simulink model "psm_svpwm_nonlinear_ctrl"  (R2026a)
settings: Solver=ode23tb  StopTime=simlength  FixedStep=tc  MaxStep=tc
values from neighbouring files (symbols this model uses):
  CTRPIFF_CLIP_RELEASE = 0.001    [init_model.m]
  dead_time_INV = 3e-6    (= 3e-06)    [init_model.m]
  emf_fb_p = 0.2    [init_model.m]
  emf_fb_p_ccaller_1 = emf_fb_p    (= 0.2)    [init_model.m]
  emf_fb_p_ccaller_2 = emf_fb_p    (= 0.2)    [init_model.m]
  emf_p = emf_fb_p*4/10    (= 0.08)    [init_model.m]
  emf_p_ccaller_1 = emf_fb_p_ccaller_1*4/10    (= 0.08)    [init_model.m]
  emf_p_ccaller_2 = emf_fb_p_ccaller_2*4/10    (= 0.08)    [init_model.m]
  fPWM_INV = fPWM_AFE    (= 5000)    [init_model.m]
  g0_10Hz = fcut_10Hz_flt * ts_afe * 2*pi    (= 0.0125663706144)    [init_model.m]
  g0_1Hz = fcut_1Hz_flt * ts_afe * 2*pi    (= 0.00125663706144)    [init_model.m]
  g1_10Hz = 1 - g0_10Hz    (= 0.987433629386)    [init_model.m]
  g1_1Hz = 1 - g0_1Hz    (= 0.998743362939)    [init_model.m]
  id_lim = 0.35    [init_model.m]
  inv_m_scale = motorc_m_scale    [init_model.m]
  iq_lim = 1.4    [init_model.m]
  kg = Kobs(1)    [init_model.m]
  ki_align = 0.1    [init_model.m]
  ki_i = 18    [init_model.m]
  ki_w = 32    [init_model.m]
  kp_align = 0.6    [init_model.m]
  kp_i = 0.25    [init_model.m]
  kp_w = 2    [init_model.m]
  kw = Kobs(2)    [init_model.m]
  lim_down_align = -0.2    [init_model.m]
  lim_up_align = 0.2    [init_model.m]
  number_of_modules = 1    [init_model.m]
  omega_m_sim = omega_m_bez    [init_model.m]
  simlength = 2    [init_model.m]
  tc = ts_afe/100    (= 2e-06)    [init_model.m]
  time_gain_afe_module_1 = 1.0    (= 1)    [init_model.m]
  time_gain_inv_module_2 = 1.0    (= 1)    [init_model.m]
  time_start_motor_control = 0.025    [init_model.m]
  ts_inv = 1/fPWM_INV    (= 0.0002)    [init_model.m]
undefined symbols (not defined in the file or in its folder): ibez, La, Lb, Ld_norm, Lq_norm, Ls_norm, magnitude, omega_bez, omega_m_bez, psi_bez, psi_m, psi_m_norm, rpm_base, rpm_bez, Rs, Rs_norm, tau_bez, torque_base, ubez
libraries: fl_lib x24, nesl_utility x11, cstblocks_lti x2, single_phase_pwm_modulator x1, pi_ctrl x1, threephase_inductor_lib x1, simple_flexible_shaft x1, permanent_magnet_synchronous_machine x1
(part 2 of 3)

== system psm_svpwm_nonlinear_ctrl/inv_psm_mod1/inverter_ctrl/inverter_control/current_ctrl/bemf_observer ==
  ialpha_pu : Inport
  ibeta_pu : Inport  Port=2
  ualpha_pu : Inport  Port=3
  ubeta_pu : Inport  Port=4
  udc_pu : Inport  Port=5
  BEMF Observer simulink/Ccaller mod1 : Scope  NumInputPorts=2
      settings: ActiveDisplayYMinimum=-0.23480320261212159  ActiveDisplayYMaximum=2.113226231053849
  Mux : Mux  Inputs=3
  Mux1 : Mux  Inputs=3
  Variant Source : VariantSource  VariantControls={use_observer_from_simulink_module_1 == 1, use_observer_from_ccaller_module_1 == 1}
  Variant Source1 : VariantSource  VariantControls={use_observer_from_simulink_module_1 == 1, use_observer_from_ccaller_module_1 == 1}
  bemf_observer : Subsystem  Commented=on
  bemf_observer_ccaller : Subsystem
  nonlinear_observer : Subsystem
  tag scope: omega_hat_pu_mod1=scoped, phase_hat_mod1=scoped
  wires:
  ialpha_pu/1 -> bemf_observer_ccaller/1(ialpha_pu), nonlinear_observer/1(ialpha_pu)
  ibeta_pu/1 -> bemf_observer_ccaller/2(ibeta_pu), nonlinear_observer/2(ibeta_pu)
  Mux/1 -> BEMF Observer simulink/Ccaller mod1/1
  Mux1/1 -> BEMF Observer simulink/Ccaller mod1/2
  ualpha_pu/1 -> bemf_observer_ccaller/3(ualpha_pu), nonlinear_observer/3(ualpha_pu)
  ubeta_pu/1 -> bemf_observer_ccaller/4(ubeta_pu), nonlinear_observer/4(ubeta_pu)
  bemf_observer_ccaller/2(theta_hat) -> Mux1/2, Variant Source1/2  "theta_hat_code"
  bemf_observer_ccaller/1(omega_pu) -> Mux/2, Variant Source/2  "omega_pu_code"
  Variant Source1/1 -> [phase_hat_mod1]
  Variant Source/1 -> [omega_hat_pu_mod1]
  udc_pu/1 -> bemf_observer_ccaller/5(udc_pu), nonlinear_observer/5(udc_pu)
  [omega_pu_psm] -> Mux/3  "omega_pu_psm_encoder"
  [phased_psm] -> Mux1/3  "phase_psm_encoder"
  [theta_z_hat] -> Variant Source1/1
  [omega_z_pu_hat] -> Variant Source/1
  [omega_z_pu_hat] -> Mux/1
  [theta_z_hat] -> Mux1/1

== system psm_svpwm_nonlinear_ctrl/inv_psm_mod1/inverter_ctrl/inverter_control/current_ctrl/current_ctrl ==
  iq_ref : Inport
  udc_pu : Inport  Port=2
  MTPA _mod1 : Subsystem
  Sqrt : Sqrt
  Square : Math  Operator=square
  Square1 : Math  Operator=square
  Sum : Sum  Inputs=|++
  dq_pi_with_vector_antiwindup mod1 : Subsystem
  id_ref _mod1 : Subsystem
      settings: PortSchema="{\"entries\":[{\"content\":{\"sides\":[{\"content\":{},\"type\":\"ConnectorPlacement.EquallySpacedRectSide\",\"uuid\":\"42af5d69-f0eb-42c6-9e03-28c1d0757323\"},{\"content\":{\"connectorIds\":[\"Out1\"],\"side\":\"RIGHT\"},\"type\":\"ConnectorPlacement.EquallySpacedRectSide\",\"uuid\":\"dd68a9f9-d15f-4e57-9d9e-130889a7b90c\"},{\"content\":{\"connectorIds\":[\"In1\"],\"side\":\"TOP\"},\"type\":\"ConnectorPlacement.EquallySpacedRectSide\",\"uuid\":\"68c797a2-8439-4b8d-8368-b7485adf0676\"}]},\"type\":\"ConnectorPlacement.EquallySpacedConnector\",\"uuid\":\"693c5f1c-0580-4626-8f13-b27865dfb3ac\"}],\"packageUris\":[\"http://schema.mathworks.com/mf0/Connector/R2020b\"],\"version\":\"1.0\"}"
  idref/id mod1 : Scope  NumInputPorts=2
      settings: ActiveDisplayYMinimum=-1.4397848868479775  ActiveDisplayYMaximum=0.32158973081029762
  iqref/iq mod1 : Scope  NumInputPorts=2
      settings: ActiveDisplayYMinimum=-1.2112726866098484  ActiveDisplayYMaximum=0.690933447736122  DataLoggingVariableName=ScopeData2
  output voltage transformation : Subsystem
  tag scope: id_pu_ref_mod1=scoped, iq_pu_ref_mod1=scoped, u_mot_pu_mod1=scoped, ud_pu_mod1=scoped, uq_pu_mod1=scoped
  wires:
  [iq_pu_mod1] -> iqref/iq mod1/2, dq_pi_with_vector_antiwindup mod1/4(iq)  "iq"
  [id_pu_mod1] -> idref/id mod1/2, dq_pi_with_vector_antiwindup mod1/2(id)  "id"
  MTPA _mod1/1(Id_ref_mtpa) -> id_ref _mod1/1(id_mtpa), [id_pu_ref_mod1]  "id_ref"
  iq_ref/1 -> MTPA _mod1/1(iq_ref), iqref/iq mod1/1, dq_pi_with_vector_antiwindup mod1/3(iq_ref), [iq_pu_ref_mod1]  "iq_ref"
  dq_pi_with_vector_antiwindup mod1/1(ctrl_d_u) -> [ud_pu_mod1], Square1/1
  dq_pi_with_vector_antiwindup mod1/2(ctrl_q_u) -> [uq_pu_mod1], Square/1
  Square/1 -> Sum/1
  Sum/1 -> Sqrt/1
  Square1/1 -> Sum/2
  Sqrt/1 -> [u_mot_pu_mod1]
  id_ref _mod1/1(id_ref) -> idref/id mod1/1, dq_pi_with_vector_antiwindup mod1/1(id_ref)
  udc_pu/1 -> dq_pi_with_vector_antiwindup mod1/5(udc_pu)

== system psm_svpwm_nonlinear_ctrl/inv_psm_mod1/inverter_ctrl/inverter_control/current_ctrl/current_transformation ==
  Demux : Demux  Outputs=3
  alphabeta2dq : MATLAB Function  TreatAsAtomicUnit=on
  uvw2alphabeta : MATLAB Function  TreatAsAtomicUnit=on
  tag scope: ialpha_pu_mod1=scoped, ibeta_pu_mod1=scoped, id_pu_mod1=scoped, iq_pu_mod1=scoped
  wires:
  alphabeta2dq/2(q) -> [iq_pu_mod1]  "iq_pu"
  alphabeta2dq/1(d) -> [id_pu_mod1]  "id_pu"
  uvw2alphabeta/2(beta) -> alphabeta2dq/2(beta), [ibeta_pu_mod1]  "ibeta_pu"
  uvw2alphabeta/1(alpha) -> [ialpha_pu_mod1], alphabeta2dq/1(alpha)  "ialpha_pu"
  [motor_phase_ctrl_mod1] -> alphabeta2dq/3(gamma)
  Demux/3 -> uvw2alphabeta/3(w)  "iw"
  Demux/2 -> uvw2alphabeta/2(v)  "iv"
  Demux/1 -> uvw2alphabeta/1(u)  "iu"
  [isd_uvw_inv_mod1] -> Demux/1

== system psm_svpwm_nonlinear_ctrl/inv_psm_mod1/inverter_ctrl/inverter_control/encoder-sensorless-switch/double_integrator_observer ==
  theta_psm : Inport
  Dead Zone : DeadZone  LowerValue=-0.01  UpperValue=0.01
  Gain : Gain  Gain=kw
  Gain1 : Gain  Gain=kg
  Gain2 : Gain  Gain=omega_bez
  Gain3 : Gain  Gain=1/omega_bez
  Gain5 : Gain  Gain=ts_inv
  Sum : Sum  Inputs=-+|
  Sum1 : Sum  Inputs=|++
  Sum2 : Sum  Inputs=|++
  Sum8 : Sum  Inputs=++|
  Unit Delay1 : UnitDelay  InitialCondition=pi  SampleTime=-1
  Unit Delay2 : UnitDelay  SampleTime=-1
  bounder1 : MATLAB Function  TreatAsAtomicUnit=on
  bounder2 : MATLAB Function  TreatAsAtomicUnit=on
  phase_psm_hat : Outport  VectorParamsAs1DForOutWhenUnconnected=off
  omega_pu_psm_hat : Outport  Port=2  VectorParamsAs1DForOutWhenUnconnected=off
  wires:
  Gain1/1 -> Sum2/1
  theta_psm/1 -> Sum/2
  Sum8/1 -> Unit Delay1/1
  Unit Delay1/1 -> bounder2/1(u)
  Sum1/1 -> Unit Delay2/1
  Gain/1 -> Gain3/1
  Unit Delay2/1 -> omega_pu_psm_hat/1, Sum1/2, Gain5/1
  Sum2/1 -> Sum8/2
  bounder2/1(y) -> Sum2/2, phase_psm_hat/1, Sum/1  "phase_hat"
  bounder1/1(y) -> Gain1/1, Gain/1
  Gain2/1 -> Sum8/1
  Gain3/1 -> Sum1/1
  Gain5/1 -> Gain2/1
  Sum/1 -> bounder1/1(u)

== system psm_svpwm_nonlinear_ctrl/inv_psm_mod1/inverter_ctrl/inverter_control/is inv quantizzation and one step delay/is inv quantizzation and one step delay ==
  is_u_pu : Inport
  is_v_pu : Inport  Port=2
  is_w_pu : Inport  Port=3
  Gain3 : Gain  Gain=-1
  Gain4 : Gain  Gain=-1
  Gain5 : Gain  Gain=-1
  Quantizer : Quantizer  QuantizationInterval=adc_quantization
  Quantizer1 : Quantizer  QuantizationInterval=adc_quantization
  Quantizer2 : Quantizer  QuantizationInterval=adc_quantization
  Unit Delay : UnitDelay  SampleTime=-1
  Unit Delay1 : UnitDelay  SampleTime=-1
  Unit Delay2 : UnitDelay  SampleTime=-1
  Zero-Order Hold : ZeroOrderHold  SampleTime=-1
  Zero-Order Hold1 : ZeroOrderHold  SampleTime=-1
  Zero-Order Hold2 : ZeroOrderHold  SampleTime=-1
  isd_u_pu : Outport
  isd_v_pu : Outport  Port=2
  isd_w_pu : Outport  Port=3
  wires:
  Unit Delay/1 -> Gain3/1
  Unit Delay1/1 -> Gain4/1
  Unit Delay2/1 -> Gain5/1
  Quantizer/1 -> Unit Delay/1
  Quantizer1/1 -> Unit Delay1/1
  Quantizer2/1 -> Unit Delay2/1
  is_u_pu/1 -> Zero-Order Hold/1
  is_v_pu/1 -> Zero-Order Hold1/1
  is_w_pu/1 -> Zero-Order Hold2/1
  Gain3/1 -> isd_u_pu/1
  Gain4/1 -> isd_v_pu/1
  Gain5/1 -> isd_w_pu/1
  Zero-Order Hold/1 -> Quantizer/1
  Zero-Order Hold1/1 -> Quantizer1/1
  Zero-Order Hold2/1 -> Quantizer2/1

== system psm_svpwm_nonlinear_ctrl/inv_psm_mod1/inverter_ctrl/inverter_control/omega_pu/flt ==
  input : Inport
  Gain3 : Gain  Gain=g1_10Hz
  Gain6 : Gain  Gain=g0_10Hz
  Sum : Sum  Inputs=|++
  Unit Delay1 : UnitDelay  SampleTime=-1
  output : Outport  VectorParamsAs1DForOutWhenUnconnected=off
  wires:
  Gain6/1 -> Sum/1
  input/1 -> Gain6/1
  Unit Delay1/1 -> Gain3/1
  Gain3/1 -> Sum/2
  Sum/1 -> Unit Delay1/1, output/1

== system psm_svpwm_nonlinear_ctrl/inv_psm_mod1/inverter_ctrl/inverter_control/phase_compensation_1/alignment_ctrl ==
  local_time : Inport
  master_time : Inport  Port=2
  Constant : Constant  Value=0
  Gain : Gain  Gain=-1
  Sum : Sum  Inputs=|+-
  pi : Subsystem  mask{kp=kp_align, ki=ki_align, lim_up=lim_up_align, lim_down=lim_down_align}
      mask prompts: ki "ki*ts"
      mask Display:
      | disp('pi()');
      | port_label('input', 1, 'u_ref');
      | port_label('input', 2, 'u');
      | port_label('output', 1, 'y');
  dp : Outport
  wires:
  master_time/1 -> Sum/1
  Sum/1 -> Gain/1
  Constant/1 -> pi/1(u_ref)
  local_time/1 -> Sum/2
  Gain/1 -> pi/2(u)
  pi/1(y) -> dp/1

== system psm_svpwm_nonlinear_ctrl/inv_psm_mod1/inverter_ctrl/inverter_control/speed_reference_generator/flt ==
  input : Inport
  Gain3 : Gain  Gain=g1_1Hz
  Gain6 : Gain  Gain=g0_1Hz
  Sum : Sum  Inputs=|++
  Unit Delay1 : UnitDelay  SampleTime=-1
  output : Outport  VectorParamsAs1DForOutWhenUnconnected=off
  wires:
  Gain6/1 -> Sum/1
  input/1 -> Gain6/1
  Unit Delay1/1 -> Gain3/1
  Gain3/1 -> Sum/2
  Sum/1 -> Unit Delay1/1, output/1

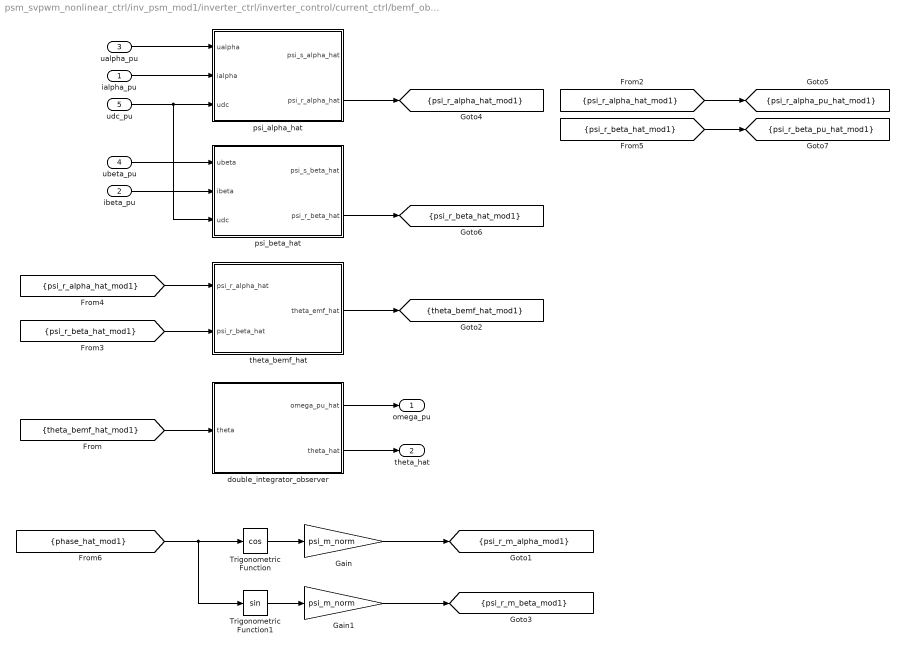
== system psm_svpwm_nonlinear_ctrl/inv_psm_mod1/inverter_ctrl/inverter_control/current_ctrl/bemf_observer/bemf_observer ==
  ialpha_pu : Inport
  ibeta_pu : Inport  Port=2
  ualpha_pu : Inport  Port=3
  ubeta_pu : Inport  Port=4
  udc_pu : Inport  Port=5
  Gain : Gain  Gain=psi_m_norm
  Gain1 : Gain  Gain=psi_m_norm
  Trigonometric Function : Trigonometry  Operator=cos
  Trigonometric Function1 : Trigonometry
  double_integrator_observer : Subsystem
  psi_alpha_hat : Subsystem
  psi_beta_hat : Subsystem
  theta_bemf_hat : Subsystem
  omega_pu : Outport
  theta_hat : Outport  Port=2
  tag scope: psi_r_alpha_hat_mod1=scoped, psi_r_alpha_pu_hat_mod1=scoped, psi_r_beta_hat_mod1=scoped, psi_r_beta_pu_hat_mod1=scoped, psi_r_m_alpha_mod1=scoped, psi_r_m_beta_mod1=scoped, theta_bemf_hat_mod1=scoped
  wires:
  Trigonometric Function/1 -> Gain/1
  Trigonometric Function1/1 -> Gain1/1
  ialpha_pu/1 -> psi_alpha_hat/2(ialpha)
  ibeta_pu/1 -> psi_beta_hat/2(ibeta)
  psi_alpha_hat/2(psi_r_alpha_hat) -> [psi_r_alpha_hat_mod1]
  psi_beta_hat/2(psi_r_beta_hat) -> [psi_r_beta_hat_mod1]
  [psi_r_alpha_hat_mod1] -> theta_bemf_hat/1(psi_r_alpha_hat)
  [psi_r_beta_hat_mod1] -> theta_bemf_hat/2(psi_r_beta_hat)
  ualpha_pu/1 -> psi_alpha_hat/1(ualpha)
  ubeta_pu/1 -> psi_beta_hat/1(ubeta)
  [phase_hat_mod1] -> Trigonometric Function/1, Trigonometric Function1/1
  Gain/1 -> [psi_r_m_alpha_mod1]
  Gain1/1 -> [psi_r_m_beta_mod1]
  theta_bemf_hat/1(theta_emf_hat) -> [theta_bemf_hat_mod1]
  [theta_bemf_hat_mod1] -> double_integrator_observer/1(theta)
  double_integrator_observer/1(omega_pu_hat) -> omega_pu/1
  double_integrator_observer/2(theta_hat) -> theta_hat/1
  [psi_r_alpha_hat_mod1] -> [psi_r_alpha_pu_hat_mod1]
  [psi_r_beta_hat_mod1] -> [psi_r_beta_pu_hat_mod1]
  udc_pu/1 -> psi_beta_hat/3(udc), psi_alpha_hat/3(udc)

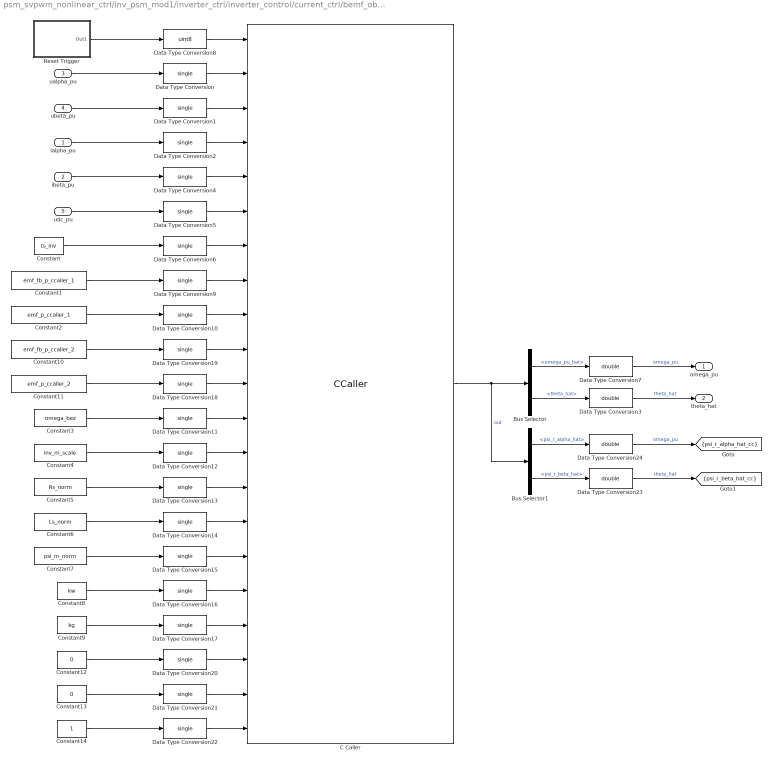
== system psm_svpwm_nonlinear_ctrl/inv_psm_mod1/inverter_ctrl/inverter_control/current_ctrl/bemf_observer/bemf_observer_ccaller ==
  ialpha_pu : Inport
  ibeta_pu : Inport  Port=2
  ualpha_pu : Inport  Port=3
  ubeta_pu : Inport  Port=4
  udc_pu : Inport  Port=5
  Bus Selector : BusSelector  OutputSignals=omega_pu_hat,theta_hat
  Bus Selector1 : BusSelector  OutputSignals=psi_r_alpha_hat,psi_r_beta_hat
  C Caller : CCaller  FunctionName=bemf_obsv_process_simulink  PortSpecificationStruct="%)30     .    N\"8   8    (     @         %    \"    !8    !     0         %  0 \"0    $    _    07)G3F%M90  4&]R=$YA;64 4V-O<&4     26YD97@     5'EP90      4VEZ90      27-';&]B86P   X    P    !@    @    $          4    (     0    ,    !         !   P!O=70 #@   #     &    \"     0         !0    @    !     P    $         $  # &]U=  .    .     8    (    !          %    \"     $    &     0         0  ...(+12985 chars)"
  Constant : Constant  Value=ts_inv
  Constant1 : Constant  Value=emf_fb_p_ccaller_1
  Constant10 : Constant  Value=emf_fb_p_ccaller_2
  Constant11 : Constant  Value=emf_p_ccaller_2
  Constant12 : Constant  Value=0
  Constant13 : Constant  Value=0
  Constant14 : Constant
  Constant2 : Constant  Value=emf_p_ccaller_1
  Constant3 : Constant  Value=omega_bez
  Constant4 : Constant  Value=inv_m_scale
  Constant5 : Constant  Value=Rs_norm
  Constant6 : Constant  Value=Ls_norm
  Constant7 : Constant  Value=psi_m_norm
  Constant8 : Constant  Value=kw
  Constant9 : Constant  Value=kg
  Data Type Conversion{,1..2,4..6,9..22} (20 alike) : DataTypeConversion  OutDataTypeStr=single  SaturateOnIntegerOverflow=off  RndMeth=Floor
  Data Type Conversion{3,7,23..24} (4 alike) : DataTypeConversion  OutDataTypeStr=double  SaturateOnIntegerOverflow=off  RndMeth=Floor
  Data Type Conversion8 : DataTypeConversion  OutDataTypeStr=uint8  SaturateOnIntegerOverflow=off  RndMeth=Floor
  Reset Trigger : Subsystem
  omega_pu : Outport
  theta_hat : Outport  Port=2
  tag scope: psi_r_alpha_hat_cc=scoped, psi_r_beta_hat_cc=scoped
  wires:
  Data Type Conversion5/1 -> C Caller/6
  Data Type Conversion/1 -> C Caller/2
  C Caller/1 -> Bus Selector1/1, Bus Selector/1  "out"
  Data Type Conversion1/1 -> C Caller/3
  Data Type Conversion4/1 -> C Caller/5
  Data Type Conversion2/1 -> C Caller/4
  Data Type Conversion6/1 -> C Caller/7
  Bus Selector/2 -> Data Type Conversion3/1  "<theta_hat>"
  Bus Selector/1 -> Data Type Conversion7/1  "<omega_pu_hat>"
  Data Type Conversion7/1 -> omega_pu/1  "omega_pu"
  Data Type Conversion3/1 -> theta_hat/1  "theta_hat"
  Data Type Conversion8/1 -> C Caller/1
  Data Type Conversion9/1 -> C Caller/8
  Data Type Conversion10/1 -> C Caller/9
  Data Type Conversion19/1 -> C Caller/10
  Data Type Conversion18/1 -> C Caller/11
  Data Type Conversion11/1 -> C Caller/12
  Data Type Conversion12/1 -> C Caller/13
  Data Type Conversion13/1 -> C Caller/14
  Data Type Conversion14/1 -> C Caller/15
  Data Type Conversion15/1 -> C Caller/16
  Data Type Conversion16/1 -> C Caller/17
  Data Type Conversion17/1 -> C Caller/18
  Data Type Conversion20/1 -> C Caller/19
  Data Type Conversion21/1 -> C Caller/20
  Data Type Conversion22/1 -> C Caller/21
  Constant14/1 -> Data Type Conversion22/1
  Constant13/1 -> Data Type Conversion21/1
  Constant12/1 -> Data Type Conversion20/1
  Constant9/1 -> Data Type Conversion17/1
  Constant8/1 -> Data Type Conversion16/1
  Constant7/1 -> Data Type Conversion15/1
  Constant6/1 -> Data Type Conversion14/1
  Constant5/1 -> Data Type Conversion13/1
  Constant4/1 -> Data Type Conversion12/1
  Constant3/1 -> Data Type Conversion11/1
  Constant11/1 -> Data Type Conversion18/1
  Constant10/1 -> Data Type Conversion19/1
  Constant2/1 -> Data Type Conversion10/1
  Constant1/1 -> Data Type Conversion9/1
  Constant/1 -> Data Type Conversion6/1
  ibeta_pu/1 -> Data Type Conversion4/1
  ialpha_pu/1 -> Data Type Conversion2/1
  ubeta_pu/1 -> Data Type Conversion1/1
  ualpha_pu/1 -> Data Type Conversion/1
  Reset Trigger/1(Out1) -> Data Type Conversion8/1
  udc_pu/1 -> Data Type Conversion5/1
  Data Type Conversion23/1 -> [psi_r_beta_hat_cc]  "theta_hat"
  Data Type Conversion24/1 -> [psi_r_alpha_hat_cc]  "omega_pu"
  Bus Selector1/1 -> Data Type Conversion24/1  "<psi_r_alpha_hat>"
  Bus Selector1/2 -> Data Type Conversion23/1  "<psi_r_beta_hat>"

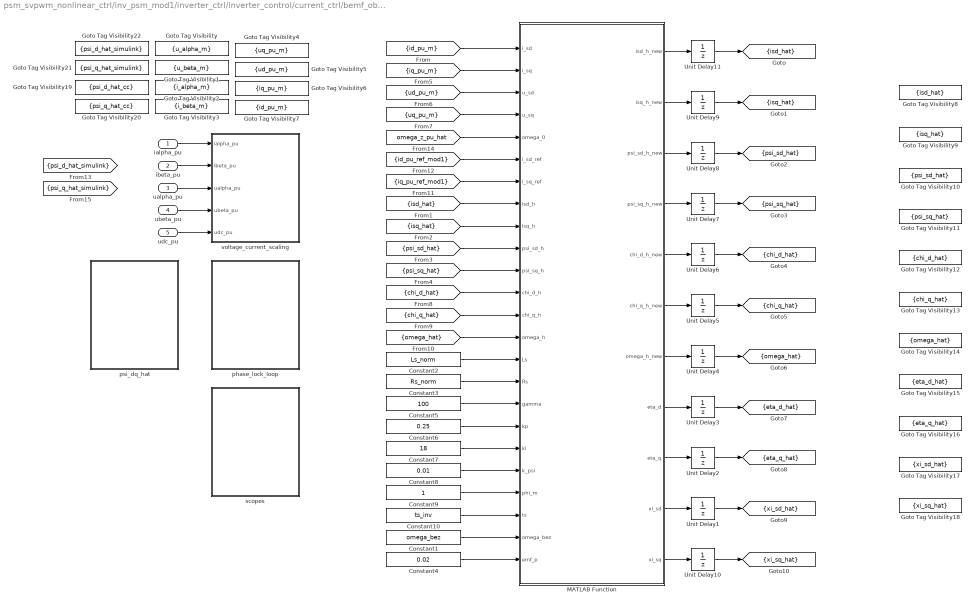
== system psm_svpwm_nonlinear_ctrl/inv_psm_mod1/inverter_ctrl/inverter_control/current_ctrl/bemf_observer/nonlinear_observer ==
  ialpha_pu : Inport
  ibeta_pu : Inport  Port=2
  ualpha_pu : Inport  Port=3
  ubeta_pu : Inport  Port=4
  udc_pu : Inport  Port=5
  Constant1 : Constant  Value=omega_bez
  Constant10 : Constant  Value=ts_inv
  Constant2 : Constant  Value=Ls_norm
  Constant3 : Constant  Value=Rs_norm
  Constant4 : Constant  Value=0.02
  Constant5 : Constant  Value=100
  Constant6 : Constant  Value=0.25
  Constant7 : Constant  Value=18
  Constant8 : Constant  Value=0.01
  Constant9 : Constant
  Goto Tag Visibility : GotoTagVisibility  GotoTag=u_alpha_m
  Goto Tag Visibility1 : GotoTagVisibility  GotoTag=u_beta_m
  Goto Tag Visibility10 : GotoTagVisibility  GotoTag=psi_sd_hat
  Goto Tag Visibility11 : GotoTagVisibility  GotoTag=psi_sq_hat
  Goto Tag Visibility12 : GotoTagVisibility  GotoTag=chi_d_hat
  Goto Tag Visibility13 : GotoTagVisibility  GotoTag=chi_q_hat
  Goto Tag Visibility14 : GotoTagVisibility  GotoTag=omega_hat
  Goto Tag Visibility15 : GotoTagVisibility  GotoTag=eta_d_hat
  Goto Tag Visibility16 : GotoTagVisibility  GotoTag=eta_q_hat
  Goto Tag Visibility17 : GotoTagVisibility  GotoTag=xi_sd_hat
  Goto Tag Visibility18 : GotoTagVisibility  GotoTag=xi_sq_hat
  Goto Tag Visibility19 : GotoTagVisibility  GotoTag=psi_d_hat_cc
  Goto Tag Visibility2 : GotoTagVisibility  GotoTag=i_alpha_m
  Goto Tag Visibility20 : GotoTagVisibility  GotoTag=psi_q_hat_cc
  Goto Tag Visibility21 : GotoTagVisibility  GotoTag=psi_q_hat_simulink
  Goto Tag Visibility22 : GotoTagVisibility  GotoTag=psi_d_hat_simulink
  Goto Tag Visibility3 : GotoTagVisibility  GotoTag=i_beta_m
  Goto Tag Visibility4 : GotoTagVisibility  GotoTag=uq_pu_m
  Goto Tag Visibility5 : GotoTagVisibility  GotoTag=ud_pu_m
  Goto Tag Visibility6 : GotoTagVisibility  GotoTag=iq_pu_m
  Goto Tag Visibility7 : GotoTagVisibility  GotoTag=id_pu_m
  Goto Tag Visibility8 : GotoTagVisibility  GotoTag=isd_hat
  Goto Tag Visibility9 : GotoTagVisibility  GotoTag=isq_hat
  MATLAB Function : MATLAB Function  TreatAsAtomicUnit=on
  Unit Delay{1..11} (11 alike) : UnitDelay  SampleTime=-1
  phase_lock_loop : Subsystem
  psi_dq_hat : Subsystem
  scopes : Subsystem
  voltage_current_scaling : Subsystem
  tag scope: chi_d_hat=scoped, chi_q_hat=scoped, eta_d_hat=scoped, eta_q_hat=scoped, isd_hat=scoped, isq_hat=scoped, omega_hat=scoped, psi_sd_hat=scoped, psi_sq_hat=scoped, xi_sd_hat=scoped, xi_sq_hat=scoped
  wires:
  ialpha_pu/1 -> voltage_current_scaling/1(ialpha_pu)
  ibeta_pu/1 -> voltage_current_scaling/2(ibeta_pu)
  ualpha_pu/1 -> voltage_current_scaling/3(ualpha_pu)
  ubeta_pu/1 -> voltage_current_scaling/4(ubeta_pu)
  udc_pu/1 -> voltage_current_scaling/5(udc_pu)
  [iq_pu_m] -> MATLAB Function/2(i_sq)
  [id_pu_m] -> MATLAB Function/1(i_sd)
  [ud_pu_m] -> MATLAB Function/3(u_sd)
  [uq_pu_m] -> MATLAB Function/4(u_sq)
  [id_pu_ref_mod1] -> MATLAB Function/6(i_sd_ref)
  [iq_pu_ref_mod1] -> MATLAB Function/7(i_sq_ref)
  MATLAB Function/1(isd_h_new) -> Unit Delay11/1
  Unit Delay11/1 -> [isd_hat]
  Unit Delay9/1 -> [isq_hat]
  MATLAB Function/2(isq_h_new) -> Unit Delay9/1
  MATLAB Function/4(psi_sq_h_new) -> Unit Delay7/1
  Unit Delay7/1 -> [psi_sq_hat]
  Unit Delay8/1 -> [psi_sd_hat]
  MATLAB Function/3(psi_sd_h_new) -> Unit Delay8/1
  Unit Delay6/1 -> [chi_d_hat]
  Unit Delay5/1 -> [chi_q_hat]
  MATLAB Function/5(chi_d_h_new) -> Unit Delay6/1
  MATLAB Function/6(chi_q_h_new) -> Unit Delay5/1
  MATLAB Function/10(xi_sd) -> Unit Delay1/1
  MATLAB Function/9(eta_q) -> Unit Delay2/1
  Unit Delay1/1 -> [xi_sd_hat]
  Unit Delay2/1 -> [eta_q_hat]
  MATLAB Function/7(omega_h_new) -> Unit Delay4/1
  Unit Delay4/1 -> [omega_hat]
  Unit Delay3/1 -> [eta_d_hat]
  MATLAB Function/8(eta_d) -> Unit Delay3/1
  Unit Delay10/1 -> [xi_sq_hat]
  MATLAB Function/11(xi_sq) -> Unit Delay10/1
  [isd_hat] -> MATLAB Function/8(isd_h)
  [isq_hat] -> MATLAB Function/9(isq_h)
  [chi_d_hat] -> MATLAB Function/12(chi_d_h)
  [chi_q_hat] -> MATLAB Function/13(chi_q_h)
  [omega_hat] -> MATLAB Function/14(omega_h)
  Constant2/1 -> MATLAB Function/15(Ls)
  [omega_z_pu_hat] -> MATLAB Function/5(omega_0)
  Constant3/1 -> MATLAB Function/16(Rs)
  Constant5/1 -> MATLAB Function/17(gamma)
  Constant6/1 -> MATLAB Function/18(kp)
  Constant7/1 -> MATLAB Function/19(ki)
  Constant8/1 -> MATLAB Function/20(k_psi)
  Constant9/1 -> MATLAB Function/21(phi_m)
  Constant10/1 -> MATLAB Function/22(ts)
  Constant1/1 -> MATLAB Function/23(omega_bez)
  [psi_sd_hat] -> MATLAB Function/10(psi_sd_h)
  [psi_sq_hat] -> MATLAB Function/11(psi_sq_h)
  Constant4/1 -> MATLAB Function/24(emf_p)

== system psm_svpwm_nonlinear_ctrl/inv_psm_mod1/inverter_ctrl/inverter_control/current_ctrl/current_ctrl/MTPA _mod1 ==
  iq_ref : Inport
  Gain1 : Gain  Gain=1/(Ld_norm - Lq_norm)/2
  Gain2 : Gain  Gain=1/(Ld_norm - Lq_norm)/2
  Gain3 : Gain  Gain=-1
  Math Function1 : Math  Operator=magnitude^2  SignedPower=on
  Math Function4 : Math  Operator=magnitude^2  SignedPower=on
  Sqrt : Sqrt
  Sum : Sum  Inputs=|++
  Sum1 : Sum  Inputs=|-+
  id_ref_pu < x < 0 : Saturate  UpperLimit=0  LowerLimit=-id_lim
  Id_ref_mtpa : Outport  VectorParamsAs1DForOutWhenUnconnected=off
  wires:
  Sum1/1 -> Gain3/1
  id_ref_pu < x < 0/1 -> Id_ref_mtpa/1
  Math Function4/1 -> Sum/1
  Math Function1/1 -> Sum/2
  Gain1/1 -> Math Function4/1
  Sum/1 -> Sqrt/1
  Sqrt/1 -> Sum1/2
  iq_ref/1 -> Math Function1/1
  Gain2/1 -> Sum1/1
  [motor_speed_pu_ctrl_mod1] -> Gain1/1, Gain2/1
  Gain3/1 -> id_ref_pu < x < 0/1

== system psm_svpwm_nonlinear_ctrl/inv_psm_mod1/inverter_ctrl/inverter_control/current_ctrl/current_ctrl/dq_pi_with_vector_antiwindup mod1 ==
  id_ref : Inport
  id : Inport  Port=2
  iq_ref : Inport  Port=3
  iq : Inport  Port=4
  udc_pu : Inport  Port=5
  Variant Source : VariantSource  VariantControls={use_current_controller_from_simulink_module_1 == 1, use_current_controller_from_ccaller_module_1 == 1}
  Variant Source1 : VariantSource  VariantControls={use_current_controller_from_simulink_module_1 == 1, use_current_controller_from_ccaller_module_1 == 1}
  dq_vector_pi : Subsystem
  dq_vector_pi_ccaller : Subsystem
  simulink/Ccaller VectorPI : Scope  NumInputPorts=2
      settings: ActiveDisplayYMinimum=-0.21776539832353589  ActiveDisplayYMaximum=0.88052476197481155
  ctrl_d_u : Outport
  ctrl_q_u : Outport  Port=2
  wires:
  id/1 -> dq_vector_pi_ccaller/1(id), dq_vector_pi/1(id)  "id"
  id_ref/1 -> dq_vector_pi_ccaller/2(id_ref), dq_vector_pi/2(id_ref)  "id_ref"
  iq/1 -> dq_vector_pi_ccaller/3(iq), dq_vector_pi/3(iq)  "iq"
  iq_ref/1 -> dq_vector_pi_ccaller/4(iq_ref), dq_vector_pi/4(iq_ref)  "iq_ref"
  dq_vector_pi/1(md_sat) -> Variant Source/1
  dq_vector_pi_ccaller/2(uq_ctrl_out) -> Variant Source1/2
  dq_vector_pi/2(mq_sat) -> Variant Source1/1
  dq_vector_pi_ccaller/1(ud_ctrl_out) -> Variant Source/2
  Variant Source/1 -> ctrl_d_u/1, simulink/Ccaller VectorPI/1  "ctrl_d_u"
  Variant Source1/1 -> simulink/Ccaller VectorPI/2, ctrl_q_u/1  "ctrl_q_u"
  udc_pu/1 -> dq_vector_pi_ccaller/5(udc_pu)

== system psm_svpwm_nonlinear_ctrl/inv_psm_mod1/inverter_ctrl/inverter_control/current_ctrl/current_ctrl/id_ref _mod1 ==
  id_mtpa : Inport
  Constant : Constant  Value=0
  Variant Source : VariantSource  VariantControls={use_mtpa == 1, use_mtpa == 0}
  id_ref : Outport
  wires:
  Variant Source/1 -> id_ref/1
  id_mtpa/1 -> Variant Source/1
  Constant/1 -> Variant Source/2

== system psm_svpwm_nonlinear_ctrl/inv_psm_mod1/inverter_ctrl/inverter_control/current_ctrl/current_ctrl/output voltage transformation ==
  Unit Delay2 : UnitDelay  SampleTime=-1
  Unit Delay3 : UnitDelay  SampleTime=-1
  dq2alphabeta : MATLAB Function  TreatAsAtomicUnit=on
  tag scope: ualpha_pu_mod1=scoped, ubeta_pu_mod1=scoped
  wires:
  [ud_pu_mod1] -> dq2alphabeta/1(d)
  [uq_pu_mod1] -> dq2alphabeta/2(q)
  Unit Delay2/1 -> [ualpha_pu_mod1]
  dq2alphabeta/2(beta) -> Unit Delay3/1
  Unit Delay3/1 -> [ubeta_pu_mod1]
  dq2alphabeta/1(alpha) -> Unit Delay2/1
  [motor_phase_ctrl_mod1] -> dq2alphabeta/3(gamma)

== system psm_svpwm_nonlinear_ctrl/inv_psm_mod1/inverter_ctrl/inverter_control/phase_compensation_1/alignment_ctrl/pi ==
  u_ref : Inport
  u : Inport  Port=2
  1/Ti : Gain  Gain=kp  SaturateOnIntegerOverflow=on  OutDataTypeStr=Inherit: Same as input  ParamDataTypeStr=Inherit: Same as input
  Saturation : Saturate  UpperLimit=lim_up  LowerLimit=lim_down
  Sum1 : Sum  Inputs=+++  SaturateOnIntegerOverflow=on
  Sum2 : Sum  Inputs=-+  SaturateOnIntegerOverflow=on
  Sum3 : Sum  Inputs=-+  SaturateOnIntegerOverflow=on
  Unit Delay4 : UnitDelay  SampleTime=-1
  kp : Gain  Gain=ki  SaturateOnIntegerOverflow=on  OutDataTypeStr=Inherit: Same as input  ParamDataTypeStr=Inherit: Same as input
  y : Outport
  wires:
  1/Ti/1 -> Sum1/1, Sum3/1
  kp/1 -> Sum1/2
  Sum3/1 -> Unit Delay4/1
  Unit Delay4/1 -> Sum1/3
  u_ref/1 -> Sum2/2
  u/1 -> Sum2/1
  Sum2/1 -> kp/1, 1/Ti/1
  Sum1/1 -> Saturation/1
  Saturation/1 -> Sum3/2, y/1

== system psm_svpwm_nonlinear_ctrl/inv_psm_mod1/inverter_ctrl/inverter_control/current_ctrl/bemf_observer/bemf_observer/double_integrator_observer ==
  theta : Inport
  Dead Zone : DeadZone  LowerValue=-0.01  UpperValue=0.01
  Gain : Gain  Gain=kw
  Gain1 : Gain  Gain=kg
  Gain2 : Gain  Gain=omega_bez
  Gain3 : Gain  Gain=1/omega_bez
  Gain5 : Gain  Gain=ts_inv
  Sum : Sum  Inputs=-+|
  Sum1 : Sum  Inputs=|++
  Sum2 : Sum  Inputs=|++
  Sum8 : Sum  Inputs=++|
  Unit Delay1 : UnitDelay  InitialCondition=pi  SampleTime=-1
  Unit Delay2 : UnitDelay  SampleTime=-1
  bounder1 : MATLAB Function  TreatAsAtomicUnit=on
  bounder2 : MATLAB Function  TreatAsAtomicUnit=on
  omega_pu_hat : Outport  VectorParamsAs1DForOutWhenUnconnected=off
  theta_hat : Outport  Port=2  VectorParamsAs1DForOutWhenUnconnected=off
  wires:
  Gain1/1 -> Sum2/1
  theta/1 -> Sum/2  "theta_bemf"
  Sum8/1 -> Unit Delay1/1
  Unit Delay1/1 -> bounder2/1(u)
  Sum1/1 -> Unit Delay2/1
  Gain/1 -> Gain3/1
  Unit Delay2/1 -> omega_pu_hat/1, Sum1/2, Gain5/1
  Sum2/1 -> Sum8/2
  bounder2/1(y) -> Sum2/2, theta_hat/1, Sum/1  "theta_hat"
  bounder1/1(y) -> Gain1/1, Gain/1
  Gain2/1 -> Sum8/1
  Gain3/1 -> Sum1/1
  Gain5/1 -> Gain2/1
  Sum/1 -> bounder1/1(u)

== system psm_svpwm_nonlinear_ctrl/inv_psm_mod1/inverter_ctrl/inverter_control/current_ctrl/bemf_observer/bemf_observer/psi_alpha_hat ==
  ualpha : Inport
  ialpha : Inport  Port=2
  udc : Inport  Port=3
  Gain1 : Gain  Gain=Rs_norm
  Gain2 : Gain  Gain=emf_fb_p
  Gain3 : Gain  Gain=emf_p
  Gain4 : Gain  Gain=omega_bez
  Gain5 : Gain  Gain=Ls_norm
  Gain6 : Gain  Gain=inv_m_scale
  Gain7 : Gain  Gain=ts_inv
  Product : Product  RndMeth=Zero
  Sum : Sum  Inputs=|+-
  Sum1 : Sum  Inputs=|+-
  Sum2 : Sum  Inputs=++-  SaturateOnIntegerOverflow=on
  Sum3 : Sum  Inputs=|++
  Sum4 : Sum  Inputs=+-  SaturateOnIntegerOverflow=on
  Unit Delay1 : UnitDelay  SampleTime=-1
  Unit Delay2 : UnitDelay  SampleTime=-1
  Unit Delay3 : UnitDelay  SampleTime=-1
  psi_s_alpha_hat : Outport  VectorParamsAs1DForOutWhenUnconnected=off
  psi_r_alpha_hat : Outport  Port=2  VectorParamsAs1DForOutWhenUnconnected=off
  wires:
  [psi_r_m_alpha_mod1] -> Sum1/1
  [psi_r_alpha_hat_mod1] -> Sum1/2
  Gain4/1 -> Gain7/1
  Sum2/1 -> Gain4/1
  Gain3/1 -> Sum2/3
  ialpha/1 -> Gain5/1, Gain1/1
  Gain1/1 -> Sum/2
  Sum/1 -> Sum2/2
  ualpha/1 -> Product/1
  Gain5/1 -> Unit Delay3/1
  Unit Delay1/1 -> Sum4/1, psi_s_alpha_hat/1, Gain3/1, Sum3/2
  Sum3/1 -> Unit Delay1/1
  Sum4/1 -> Unit Delay2/1
  Sum1/1 -> Gain2/1
  Gain2/1 -> Sum2/1
  Gain7/1 -> Sum3/1
  Product/1 -> Gain6/1
  Gain6/1 -> Sum/1
  Unit Delay2/1 -> psi_r_alpha_hat/1
  Unit Delay3/1 -> Sum4/2
  udc/1 -> Product/2

== system psm_svpwm_nonlinear_ctrl/inv_psm_mod1/inverter_ctrl/inverter_control/current_ctrl/bemf_observer/bemf_observer/psi_beta_hat ==
  ubeta : Inport
  ibeta : Inport  Port=2
  udc : Inport  Port=3
  Gain1 : Gain  Gain=Rs_norm
  Gain2 : Gain  Gain=emf_fb_p
  Gain3 : Gain  Gain=emf_p
  Gain4 : Gain  Gain=omega_bez
  Gain5 : Gain  Gain=Ls_norm
  Gain6 : Gain  Gain=inv_m_scale
  Gain7 : Gain  Gain=ts_inv
  Product : Product  RndMeth=Zero
  Sum : Sum  Inputs=|+-
  Sum1 : Sum  Inputs=|+-
  Sum2 : Sum  Inputs=++-  SaturateOnIntegerOverflow=on
  Sum3 : Sum  Inputs=|++
  Sum4 : Sum  Inputs=+-  SaturateOnIntegerOverflow=on
  Unit Delay1 : UnitDelay  SampleTime=-1
  Unit Delay2 : UnitDelay  SampleTime=-1
  Unit Delay3 : UnitDelay  SampleTime=-1
  psi_s_beta_hat : Outport  VectorParamsAs1DForOutWhenUnconnected=off
  psi_r_beta_hat : Outport  Port=2  VectorParamsAs1DForOutWhenUnconnected=off
  wires:
  Gain5/1 -> Unit Delay3/1
  Sum/1 -> Sum2/2
  Gain1/1 -> Sum/2
  ibeta/1 -> Gain5/1, Gain1/1
  Gain3/1 -> Sum2/3
  Sum2/1 -> Gain4/1
  Gain4/1 -> Gain7/1
  Sum1/1 -> Gain2/1
  [psi_r_beta_hat_mod1] -> Sum1/2
  [psi_r_m_beta_mod1] -> Sum1/1
  Unit Delay1/1 -> Gain3/1, Sum4/1, psi_s_beta_hat/1, Sum3/2
  Sum3/1 -> Unit Delay1/1
  Sum4/1 -> Unit Delay2/1
  Gain2/1 -> Sum2/1
  ubeta/1 -> Product/1
  Gain7/1 -> Sum3/1
  Product/1 -> Gain6/1
  Gain6/1 -> Sum/1
  Unit Delay2/1 -> psi_r_beta_hat/1
  Unit Delay3/1 -> Sum4/2
  udc/1 -> Product/2

== system psm_svpwm_nonlinear_ctrl/inv_psm_mod1/inverter_ctrl/inverter_control/current_ctrl/bemf_observer/bemf_observer/theta_bemf_hat ==
  psi_r_alpha_hat : Inport
  psi_r_beta_hat : Inport  Port=2
  Trigonometric Function : Trigonometry  Operator=atan2  OutputSignalType=real
  theta_emf_hat : Outport  VectorParamsAs1DForOutWhenUnconnected=off
  wires:
  psi_r_alpha_hat/1 -> Trigonometric Function/2
  psi_r_beta_hat/1 -> Trigonometric Function/1
  Trigonometric Function/1 -> theta_emf_hat/1

== system psm_svpwm_nonlinear_ctrl/inv_psm_mod1/inverter_ctrl/inverter_control/current_ctrl/bemf_observer/bemf_observer_ccaller/Reset Trigger ==
  Step : Step  Time=0.01  InitialValue=1  FinalValue=0
  Out1 : Outport
  wires:
  Step/1 -> Out1/1  "Reset"

== system psm_svpwm_nonlinear_ctrl/inv_psm_mod1/inverter_ctrl/inverter_control/current_ctrl/bemf_observer/nonlinear_observer/phase_lock_loop ==
  alphabeta2dq : MATLAB Function  TreatAsAtomicUnit=on
  theta_bemf_hat : Subsystem
  tag scope: omega_z_pu_hat=global, psi_d_hat_cc=scoped, psi_q_hat_cc=scoped, theta_z_hat=global
  wires:
  theta_bemf_hat/1(omega_z) -> [omega_z_pu_hat]
  theta_bemf_hat/2(theta_z) -> [theta_z_hat]
  [omega_hat] -> theta_bemf_hat/3(omega_hat)
  [psi_r_alpha_hat_cc] -> alphabeta2dq/1(alpha)  "psi_r_alpha_hat_cc"
  [psi_r_beta_hat_cc] -> alphabeta2dq/2(beta)  "psi_r_beta_hat_cc"
  [phase_hat_mod1] -> alphabeta2dq/3(gamma)  "phase_hat_mod1"
  alphabeta2dq/1(d) -> [psi_d_hat_cc]  "id_pu"
  alphabeta2dq/2(q) -> [psi_q_hat_cc]  "iq_pu"
  [psi_sd_hat] -> theta_bemf_hat/1(psi_sd_hat)
  [psi_sq_hat] -> theta_bemf_hat/2(psi_sq_hat)

== system psm_svpwm_nonlinear_ctrl/inv_psm_mod1/inverter_ctrl/inverter_control/current_ctrl/bemf_observer/nonlinear_observer/psi_dq_hat ==
  psi_d_hat : Subsystem
  psi_q_hat : Subsystem

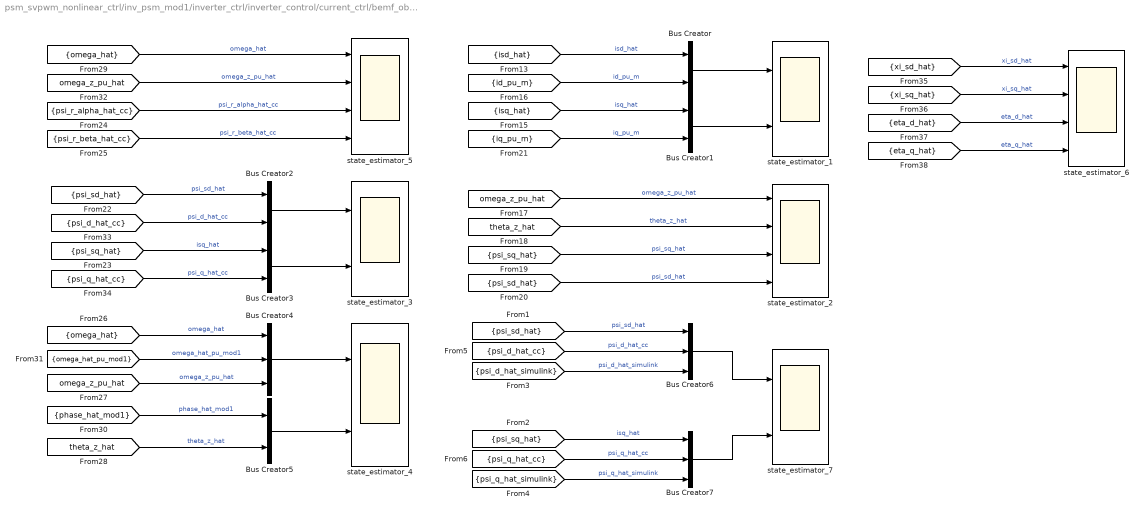
== system psm_svpwm_nonlinear_ctrl/inv_psm_mod1/inverter_ctrl/inverter_control/current_ctrl/bemf_observer/nonlinear_observer/scopes ==
  Bus Creator{,1..3,5} (5 alike) : BusCreator  Inputs=2
  Bus Creator4 : BusCreator  Inputs=3
  Bus Creator6 : BusCreator  Inputs=3
  Bus Creator7 : BusCreator  Inputs=3
  state_estimator_{1,3..4,7} (4 alike) : Scope  NumInputPorts=2
      state_estimator_1 settings: ActiveDisplayYMinimum=-1.692629590101832  ActiveDisplayYMaximum=0.74369717859211848
      state_estimator_3 settings: ActiveDisplayYMinimum=-2.6843832976750246  ActiveDisplayYMaximum=1.9911157971693669  DataLoggingVariableName=ScopeData6
      state_estimator_4 settings: ActiveDisplayYMinimum=-0.12501426116843978  ActiveDisplayYMaximum=1.125127991524423  DataLoggingVariableName=ScopeData7
      state_estimator_7 settings: ActiveDisplayYMinimum=-3.2662294119770752  ActiveDisplayYMaximum=2.4319005927819832  DataLoggingVariableName=ScopeData14
  state_estimator_2 : Scope  NumInputPorts=4
      settings: ActiveDisplayYMinimum=-0.12501639167278025  ActiveDisplayYMaximum=1.1251471660634873  DataLoggingVariableName=ScopeData4
  state_estimator_5 : Scope  NumInputPorts=4
      settings: ActiveDisplayYMinimum=-0.086851222861738325  ActiveDisplayYMaximum=0.78166064676410973  DataLoggingVariableName=ScopeData9
  state_estimator_6 : Scope  NumInputPorts=4
      settings: ActiveDisplayYMinimum=-1.4032994216885988  ActiveDisplayYMaximum=1.3085064991551667  DataLoggingVariableName=ScopeData10
  wires:
  [psi_q_hat_cc] -> Bus Creator3/2  "psi_q_hat_cc"
  [psi_r_beta_hat_cc] -> state_estimator_5/4  "psi_r_beta_hat_cc"
  Bus Creator2/1 -> state_estimator_3/1
  [omega_hat] -> state_estimator_5/1  "omega_hat"
  Bus Creator3/1 -> state_estimator_3/2
  Bus Creator5/1 -> state_estimator_4/2
  [xi_sd_hat] -> state_estimator_6/1  "xi_sd_hat"
  [omega_z_pu_hat] -> state_estimator_5/2  "omega_z_pu_hat"
  [omega_z_pu_hat] -> Bus Creator4/3  "omega_z_pu_hat"
  [omega_hat_pu_mod1] -> Bus Creator4/2  "omega_hat_pu_mod1"
  [theta_z_hat] -> Bus Creator5/2  "theta_z_hat"
  [psi_sq_hat] -> Bus Creator3/1  "isq_hat"
  [phase_hat_mod1] -> Bus Creator5/1  "phase_hat_mod1"
  [xi_sq_hat] -> state_estimator_6/2  "xi_sq_hat"
  Bus Creator4/1 -> state_estimator_4/1
  [psi_sd_hat] -> Bus Creator2/1  "psi_sd_hat"
  [eta_d_hat] -> state_estimator_6/3  "eta_d_hat"
  [psi_d_hat_cc] -> Bus Creator2/2  "psi_d_hat_cc"
  [omega_hat] -> Bus Creator4/1  "omega_hat"
  [eta_q_hat] -> state_estimator_6/4  "eta_q_hat"
  [psi_r_alpha_hat_cc] -> state_estimator_5/3  "psi_r_alpha_hat_cc"
  [iq_pu_m] -> Bus Creator1/2  "iq_pu_m"
  [psi_sd_hat] -> state_estimator_2/4  "psi_sd_hat"
  [isq_hat] -> Bus Creator1/1  "isq_hat"
  Bus Creator/1 -> state_estimator_1/1
  [omega_z_pu_hat] -> state_estimator_2/1  "omega_z_pu_hat"
  [id_pu_m] -> Bus Creator/2  "id_pu_m"
  [psi_sq_hat] -> state_estimator_2/3  "psi_sq_hat"
  Bus Creator1/1 -> state_estimator_1/2
  [isd_hat] -> Bus Creator/1  "isd_hat"
  [theta_z_hat] -> state_estimator_2/2  "theta_z_hat"
  [psi_d_hat_cc] -> Bus Creator6/2  "psi_d_hat_cc"
  [psi_sd_hat] -> Bus Creator6/1  "psi_sd_hat"
  [psi_sq_hat] -> Bus Creator7/1  "isq_hat"
  Bus Creator7/1 -> state_estimator_7/2
  Bus Creator6/1 -> state_estimator_7/1
  [psi_q_hat_cc] -> Bus Creator7/2  "psi_q_hat_cc"
  [psi_q_hat_simulink] -> Bus Creator7/3  "psi_q_hat_simulink"
  [psi_d_hat_simulink] -> Bus Creator6/3  "psi_d_hat_simulink"

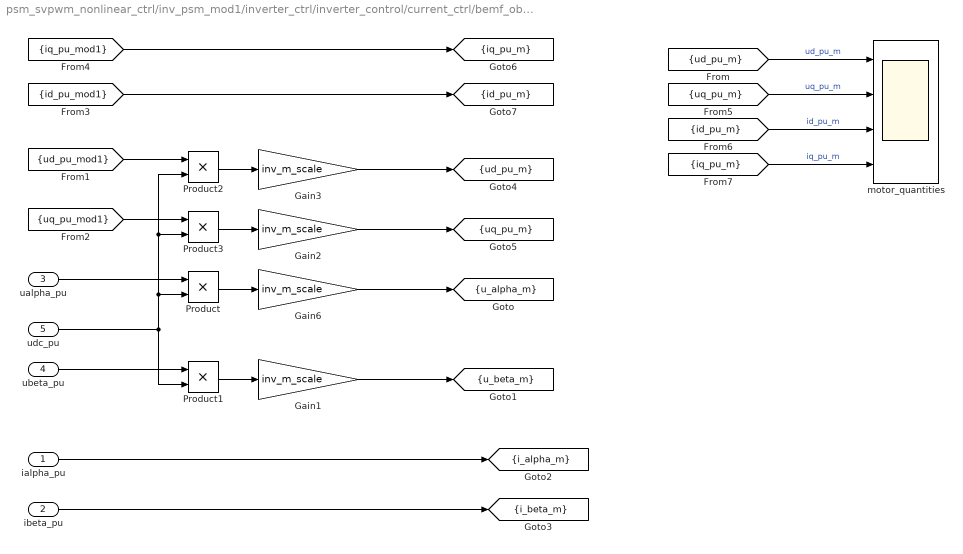
== system psm_svpwm_nonlinear_ctrl/inv_psm_mod1/inverter_ctrl/inverter_control/current_ctrl/bemf_observer/nonlinear_observer/voltage_current_scaling ==
  ialpha_pu : Inport
  ibeta_pu : Inport  Port=2
  ualpha_pu : Inport  Port=3
  ubeta_pu : Inport  Port=4
  udc_pu : Inport  Port=5
  Gain{1..3,6} (4 alike) : Gain  Gain=inv_m_scale
  Product{,1..3} (4 alike) : Product  RndMeth=Zero
  motor_quantities : Scope  NumInputPorts=4
      settings: ActiveDisplayYMinimum=-1.6203753319228322  ActiveDisplayYMaximum=1.9469037364839927  DataLoggingVariableName=ScopeData8
  tag scope: i_alpha_m=scoped, i_beta_m=scoped, id_pu_m=scoped, iq_pu_m=scoped, u_alpha_m=scoped, u_beta_m=scoped, ud_pu_m=scoped, uq_pu_m=scoped
  wires:
  [uq_pu_mod1] -> Product3/1
  [ud_pu_mod1] -> Product2/1
  ubeta_pu/1 -> Product1/1
  ualpha_pu/1 -> Product/1
  udc_pu/1 -> Product/2, Product2/2, Product3/2, Product1/2
  ialpha_pu/1 -> [i_alpha_m]
  ibeta_pu/1 -> [i_beta_m]
  Product/1 -> Gain6/1
  Product3/1 -> Gain2/1
  Product2/1 -> Gain3/1
  Product1/1 -> Gain1/1
  [ud_pu_m] -> motor_quantities/1  "ud_pu_m"
  [uq_pu_m] -> motor_quantities/2  "uq_pu_m"
  [id_pu_m] -> motor_quantities/3  "id_pu_m"
  [iq_pu_m] -> motor_quantities/4  "iq_pu_m"
  Gain3/1 -> [ud_pu_m]
  Gain2/1 -> [uq_pu_m]
  Gain6/1 -> [u_alpha_m]
  Gain1/1 -> [u_beta_m]
  [id_pu_mod1] -> [id_pu_m]
  [iq_pu_mod1] -> [iq_pu_m]
